simulink model "Bicycle_Cartesian_Regulator"  (R2024b)
settings: Solver=VariableStepAuto  StartTime=0.0  StopTime=40  RelTol=1e-3
libraries: robotmobilelib x1, sim3dlib x1, sim3dautolib x1
settings Model: Creator=loren  LastModifiedBy=loren

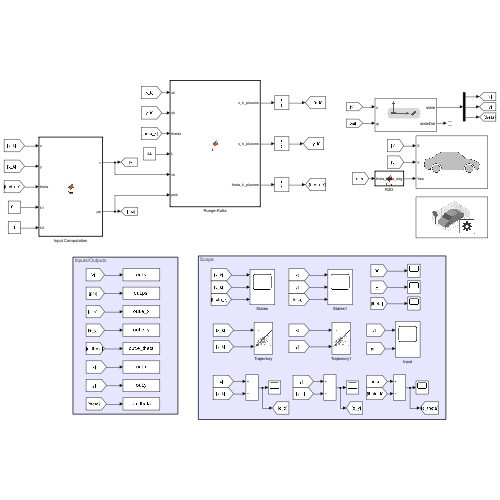
[thumbnail: Simulink's stored preview of the top-level diagram]
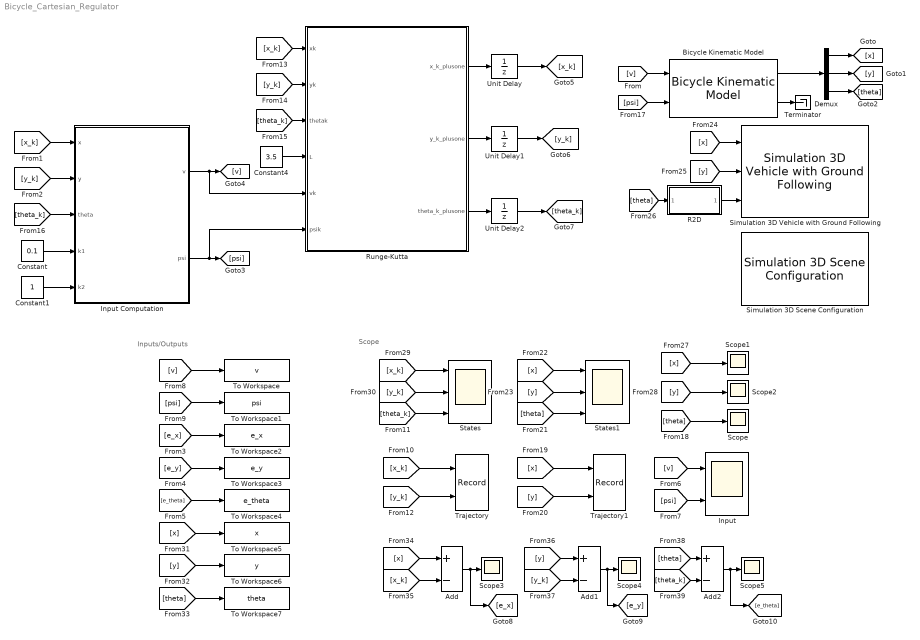
== system Bicycle_Cartesian_Regulator ==
  note: Inputs/Outputs
  note: Scope
  Add : Sum  Inputs=+-
  Add1 : Sum  Inputs=+-
  Add2 : Sum  Inputs=+-
  Bicycle Kinematic Model : robotmobilelib/Bicycle Kinematic Model  VehicleInputs=Vehicle Speed & Steering Angle  WheelBase=3.5  VehicleSpeedRange=[-inf inf]  MaxSteeringAngle=pi/3  InitialState=[-100; -50; pi/4]  SimulateUsing=Interpreted execution
  Constant : Constant  Value=0.1
  Constant1 : Constant
  Constant4 : Constant  Value=3.5
  Demux : Demux  Outputs=3
  Input : Scope  NumInputPorts=2
  Input Computation : MATLAB Function  TreatAsAtomicUnit=on
  R2D : MATLAB Function  TreatAsAtomicUnit=on
  Runge-Kutta : MATLAB Function  TreatAsAtomicUnit=on
  Scope{,1..5} (6 alike) : Scope
  Simulation 3D Scene Configuration : sim3dlib/Simulation 3D Scene Configuration  Priority=0  ProjectFormat=Default Scenes  SceneDesc=Parking lot  ProjectName=C:\Program Files\MATLAB\R2024b\toolbox\shared\sim3d_projects\automotive_project_windows\UE\WindowsNoEditor\VehicleSimulation.exe  ScenePath=/Game/Maps/HwStrght  EnableOpenDRIVE=off  vehTagList={'Custom';'Scene Origin';'SimulinkVehicle1'}  vehTag=SimulinkVehicle1  FreeCameraInitialTranslation=[0, 0, 0]  FreeCameraDefaultInitialTranslation=[-6, 0, 2]  FreeCameraInitialRotation=[0, 0, 0]  FreeCameraDefaultInitialRotation=[0, -15, 0]  OpVisEn=off  Ts=0.01  EnableWindow=on  EnableRemoteAccess=off  EnableWeather=off  SunAzimuth=90  SunAltitude=40.0  EnableGeospatialSun=off  Latitude=0  Longitude=0  Date=2023-01-01  Time=10:30:00  GeoTimeZone=-5.0  SunDaylightSaving=off  wind=1  clouds=10  EnableVolumetricClouds=off  CloudCoverage=0  CloudAltitude=6  fog=0  rain=0  RaindropsEffect=off  SnowDensity=0  EnableGeospatial=off  UseTrueOrigin=off  OriginHeight=200  OriginLatitude=40.744652  OriginLongitude=-73.988864  MapStyle=Aerial  AdditionalAssetIDs=[]  UseAdvancedSunSky=off  SolarTime=11  TimeZone=-5  Day=21  Month=9  Year=2022  UseDaylightSavingTime=on  DSTStartDay=10  DSTStartMonth=3  DSTEndDay=3  DSTEndMonth=11  DSTSwitchHour=2  sensorTag=MainCamera1  sensorId=1  sensorName=MainCamera1  mountLoc=Origin  offsetFlag=off  tmountOffset=[0, 0, 0]  rmountOffset=[0, 0, 0]  HorizontalResolution=1280  VerticalResolution=720  HorizontalFOV=60  mountPoint=[0 0 0]  mountOrientation=[0 0 0]  aMode=3  ID=1  GeoTrigger=Inactive
      settings: LibrarySourceBlock=drivingsim3d/Simulation 3D Scene Configuration
  Simulation 3D Vehicle with Ground Following : sim3dautolib/Simulation 3D Vehicle with Ground Following  Priority=-1  PassVehMesh=Muscle car  MeshPath=/MathWorksAutomotiveContent/Vehicles/Muscle/Meshes/SK_MuscleCar.SK_MuscleCar  TrackWidth=1.9  WheelBase=3  WheelRadius=0.35  VehColor=Red  InitialPos=[-100, -50, 0]  InitialRot=[0, 0, pi/4]  ActorName=SimulinkVehicle1  SampleTime=0.01  ActorType=SimulinkVehicle  ID=1  aMode=3  ActorTag=SimulinkVehicle1  CoordinateScheme=ISO  VehLightsControl=off  HeadlightColor=[ 1, 1, 1 ]  HighBeamIntensity=100000  LowBeamIntensity=60000  HighBeamConeAngle=70  LowBeamConeAngle=70  LeftHeadlightOrientation=[ 0, 0 ]  RightHeadlightOrientation=[ 0, 0 ]  BrakelightIntensity=500  ReverselightIntensity=500  SignallightIntensity=500  SignallightPeriod=1  SignalPulseWidth=50  TransformOutportEnabled=off
      settings: LibrarySourceBlock=drivingsim3d/Simulation 3D Vehicle with Ground Following
  States : Scope  NumInputPorts=3
  States1 : Scope  NumInputPorts=3
  Terminator : Terminator
  To Workspace : ToWorkspace  VariableName=v  SaveFormat=Timeseries  SampleTime=0.01
  To Workspace1 : ToWorkspace  VariableName=psi  SaveFormat=Timeseries  SampleTime=0.01
  To Workspace2 : ToWorkspace  VariableName=e_x  SaveFormat=Timeseries  SampleTime=0.01
  To Workspace3 : ToWorkspace  VariableName=e_y  SaveFormat=Timeseries  SampleTime=0.01
  To Workspace4 : ToWorkspace  VariableName=e_theta  SaveFormat=Timeseries  SampleTime=0.01
  To Workspace5 : ToWorkspace  VariableName=x  SaveFormat=Timeseries  SampleTime=0.01
  To Workspace6 : ToWorkspace  VariableName=y  SaveFormat=Timeseries  SampleTime=0.01
  To Workspace7 : ToWorkspace  VariableName=theta  SaveFormat=Timeseries  SampleTime=0.01
  Trajectory : Record  FileSettingsInternal="{\"entries\":[{\"content\":{\"excelSettings\":{\"content\":{},\"type\":\"Streamout.ExcelSettings\"}},\"type\":\"Streamout.FileSettingStorage\",\"uuid\":\"\"}],\"packageUris\":[\"http:\\/\\/schema.mathworks.com\\/mf0\\/streamout_blocks\\/R2020a\"],\"version\":\"1.0\"}"  Layout=[1 1]  SignalsInternal="{\"entries\":[{\"content\":{\"signals\":[{\"content\":{\"blockPath\":[],\"dimensions\":[1],\"domain\":\"\",\"lineColor\":\"#fe330a\",\"lineWidth\":2,\"port\":1,\"sid\":[\"\"],\"signalID\":1,\"signalName\":\"From10\"},\"type\":\"RecordBlkView.Signal\",\"uuid\":\"\"},{\"content\":{\"blockPath\":[],\"dimensions\":[1],\"domain\":\"\",\"lineColor\":\"#22b573\",\"lineWidth\":2,\"port\":2,\"sid\":[\"\"],\"signalID\":2,\"signalName\":\"From12\"},\"type\":\"RecordBlkView.Signal\",\"uuid\":\"\"}]},\"type\":\"RecordBlkView.InputSignals\",\"uuid\":\"\"}],\"packageUris\":[\"http:\\/\\/schema.mathworks.com\\/mf0\\/streamout_blocks\\/R2020a\"],\"version\":\"1.0\"}"  VisualizationBindings="{\"xyplotplugin\":{\"info\":[{\"series\":[],\"subplotID\":1}]}}"  CompatibilityTag=XY
  Trajectory1 : Record  FileSettingsInternal="{\"entries\":[{\"content\":{\"excelSettings\":{\"content\":{},\"type\":\"Streamout.ExcelSettings\"}},\"type\":\"Streamout.FileSettingStorage\",\"uuid\":\"\"}],\"packageUris\":[\"http:\\/\\/schema.mathworks.com\\/mf0\\/streamout_blocks\\/R2020a\"],\"version\":\"1.0\"}"  Layout=[1 1]  SignalsInternal="{\"entries\":[{\"content\":{\"signals\":[{\"content\":{\"blockPath\":[],\"dimensions\":[1],\"domain\":\"\",\"lineColor\":\"#a2142f\",\"plots\":[ 1 ],\"port\":1,\"sid\":[\"\"],\"signalID\":1,\"signalName\":\"From19\"},\"type\":\"RecordBlkView.Signal\",\"uuid\":\"\"},{\"content\":{\"blockPath\":[],\"dimensions\":[1],\"domain\":\"\",\"lineColor\":\"#139fff\",\"plots\":[ 1 ],\"port\":2,\"sid\":[\"\"],\"signalID\":2,\"signalName\":\"From20\"},\"type\":\"RecordBlkView.Signal\",\"uuid\":\"\"}]},\"type\":\"RecordBlkView.InputSignals\",\"uuid\":\"\"}],\"packageUris\":[\"http:\\/\\/schema.mathworks.com\\/mf0\\/streamout_blocks\\/R2020a\"],\"version\":\"1.0\"}"  VisualizationBindings="{\"xyplotplugin\":{\"info\":[{\"series\":[{\"bindingParametersList\":[{\"parameter\":\"X-Axis\",\"signalID\":1,\"signalName\":\"From19\"},{\"parameter\":\"Y-Axis\",\"signalID\":2,\"signalName\":\"From20\"}],\"seriesID\":0}],\"subplotID\":1}]}}"  CompatibilityTag=XY
  Unit Delay : UnitDelay  InitialCondition=-100  SampleTime=0.01  HasFrameUpgradeWarning=on
  Unit Delay1 : UnitDelay  InitialCondition=-50  SampleTime=0.01  HasFrameUpgradeWarning=on
  Unit Delay2 : UnitDelay  InitialCondition=pi/4  SampleTime=0.01  HasFrameUpgradeWarning=on
  wires:
  Constant/1 -> Input Computation/4(k1)
  Constant1/1 -> Input Computation/5(k2)
  Input Computation/1(v) -> Runge-Kutta/5(vk), [v]
  Input Computation/2(psi) -> Runge-Kutta/6(psik), [psi]
  Bicycle Kinematic Model/2 -> Terminator/1
  Bicycle Kinematic Model/1 -> Demux/1
  Demux/1 -> [x]
  Demux/2 -> [y]
  Demux/3 -> [theta]
  [theta_k] -> Input Computation/3(theta)
  [y_k] -> Input Computation/2(y)
  [x_k] -> Input Computation/1(x)
  [y] -> Simulation 3D Vehicle with Ground Following/2
  [x] -> Simulation 3D Vehicle with Ground Following/1
  R2D/1(theta_deg) -> Simulation 3D Vehicle with Ground Following/3
  [theta] -> R2D/1(theta_rad)
  Constant4/1 -> Runge-Kutta/4(L)
  [x_k] -> Runge-Kutta/1(xk)
  [y_k] -> Runge-Kutta/2(yk)
  [theta_k] -> Runge-Kutta/3(thetak)
  Unit Delay1/1 -> [y_k]
  Unit Delay/1 -> [x_k]
  Unit Delay2/1 -> [theta_k]
  Runge-Kutta/1(x_k_plusone) -> Unit Delay/1
  Runge-Kutta/2(y_k_plusone) -> Unit Delay1/1
  Runge-Kutta/3(theta_k_plusone) -> Unit Delay2/1
  [v] -> Bicycle Kinematic Model/1
  [theta] -> To Workspace7/1
  [psi] -> Input/2
  [theta_k] -> Add2/2
  Add/1 -> [e_x], Scope3/1
  [y] -> Add1/1
  [x] -> To Workspace5/1
  [v] -> Input/1
  [y] -> Scope2/1
  [x] -> Add/1
  [v] -> To Workspace/1
  Add1/1 -> [e_y], Scope4/1
  [x] -> Scope1/1
  [x] -> Trajectory1/1
  [x_k] -> States/1
  [y_k] -> Add1/2
  [y] -> Trajectory1/2
  [e_x] -> To Workspace2/1
  [y] -> States1/2
  [x] -> States1/1
  [y_k] -> Trajectory/2
  [theta] -> States1/3
  [psi] -> To Workspace1/1
  [y] -> To Workspace6/1
  [theta_k] -> States/3
  [x_k] -> Trajectory/1
  [y_k] -> States/2
  [e_y] -> To Workspace3/1
  [e_theta] -> To Workspace4/1
  [theta] -> Scope/1
  Add2/1 -> [e_theta], Scope5/1
  [x_k] -> Add/2
  [theta] -> Add2/1
  [psi] -> Bicycle Kinematic Model/2

== matlab function Bicycle_Cartesian_Regulator/Input Computation ==
  data: x input; y input; theta input; v output; k1 input; k2 input; psi output
function [v, psi] = fcn(x, y, theta, k1, k2)
    L = 3.5;  % Wheelbase

    % Linear Velocity
    v = - k1 * (x * cos(theta) + y * sin(theta));

    % Angular Velocity
    omega = k2 * (atan2(y,x) + pi - theta);

    % Steering Angle
    if abs(v) > 1e-6  % To avoid singularity
        psi = atan((omega * L) / v);
    else
        psi = 0;
    end

    % Maximum feasible value for psi
    psi_max = 60 * pi/180;  % ±60 degrees
    psi = max(-psi_max, min(psi_max, psi));
end

== matlab function Bicycle_Cartesian_Regulator/Runge-Kutta ==
  data: xk input; yk input; thetak input; L input; vk input; x_k_plusone output; psik input; y_k_plusone output; theta_k_plusone output
function [x_k_plusone, y_k_plusone, theta_k_plusone] = fcn(xk, yk, thetak, L, vk, psik)
    Ts = 0.01; % Sampling Time >0

    omegak = (vk / L) * tan(psik);

    x_k_plusone = xk + vk * Ts * cos(thetak + (omegak * Ts)/2);
    y_k_plusone = yk + vk * Ts * sin(thetak + (omegak * Ts)/2);
    theta_k_plusone = thetak + omegak * Ts;
end

== matlab function Bicycle_Cartesian_Regulator/R2D ==
  data: theta_rad input; theta_deg output
function theta_deg = fcn(theta_rad)

theta_deg = theta_rad*180/pi;
